simulink model "Lm35DevresiSimilunk412"  (R2015a)
settings: Solver=ode45  StartTime=0.0  StopTime=10.0  RelTol=1e-3
libraries: arduino_io_lib x4
settings Model: Creator=Osman  LastModifiedBy=Mustafa

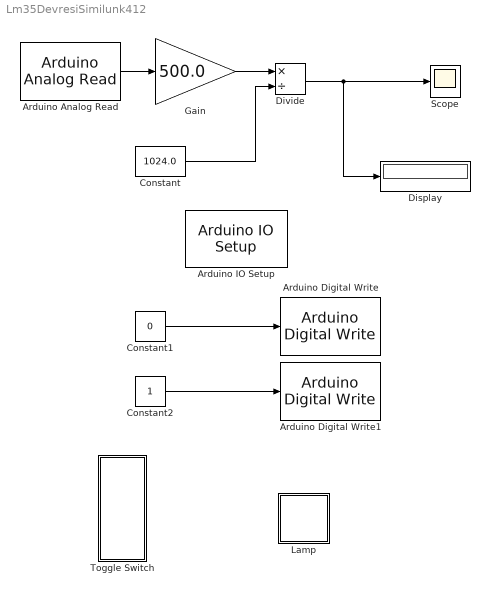
== system Lm35DevresiSimilunk412 ==
  Arduino Analog Read : arduino_io_lib/Arduino Analog Read  arduinoVar=Temporary arduino variable: Arduino1  arduinoPin=0  T=0.0001
  Arduino Digital Write : arduino_io_lib/Arduino Digital Write  arduinoVar=Temporary arduino variable: Arduino1  arduinoPin=8  T=0.2
  Arduino Digital Write1 : arduino_io_lib/Arduino Digital Write  arduinoVar=Temporary arduino variable: Arduino1  arduinoPin=7  T=0.2
  Arduino IO Setup : arduino_io_lib/Arduino IO Setup  Priority=3  arduinoVar=Temporary arduino variable: Arduino1  workspaceVarName=a  comPort=COM9
  Constant : Constant  Value=1024.0
  Constant1 : Constant  Value=0
  Constant2 : Constant
  Display : Display
  Divide : Product  Inputs=*/
  Gain : Gain  Gain=500.0
  Lamp : Subsystem  DialogController=hmiCreateDDGDialog  IsWebBlock=on  mask(MathWorksWebBlock){webBlockId=065f5afa-c7d6-415b-949f-0ad1369a6718, webBlockType=lamp, ShowInLibBrowser=on, ShowInitialText=on, HMISrcModelName=Lm35DevresiSimilunk412}
      mask prompts: webBlockType "WebBlock Type"; HMISrcModelName "Source Model"
      mask Help: helpview([docroot '/mapfiles/simulink.map'], 'hmi_lamp')
      mask Display:
      | if strcmp(get_param(bdroot(gcb),'BlockDiagramType'), 'library')
      |     image([(matlabroot) '/toolbox/simulink/hmi/icons/Lamp.png']);
      | end
  Scope : Scope
      settings: TimeRange=10  YMin=2.5  YMax=60
  Toggle Switch : Subsystem  DialogController=hmiCreateDDGDialog  IsWebBlock=on  mask(MathWorksWebBlock){webBlockId=2cad5390-662a-418e-9234-6ba5d9e14c03, webBlockType=toggleswitch, ShowInLibBrowser=on, ShowInitialText=on, HMISrcModelName=Lm35DevresiSimilunk412}
      mask prompts: webBlockId "WebBlock Id"; webBlockType "WebBlock Type"; HMISrcModelName "Source Model"
      mask Help: helpview([docroot '/mapfiles/simulink.map'], 'hmi_toggle_switch')
      mask Display:
      | if strcmp(get_param(bdroot(gcb),'BlockDiagramType'), 'library')
      |     image([(matlabroot) '/toolbox/simulink/hmi/icons/ToggleSwitch.png']);
      | end
  wires:
  Gain/1 -> Divide/1
  Constant/1 -> Divide/2
  Divide/1 -> Display/1, Scope/1
  Arduino Analog Read/1 -> Gain/1
  Constant2/1 -> Arduino Digital Write1/1
  Constant1/1 -> Arduino Digital Write/1

== system Lm35DevresiSimilunk412/Lamp ==

== system Lm35DevresiSimilunk412/Toggle Switch ==
